simulink model "exo2_Part3_y"  (R2020b)
settings: Solver=VariableStepAuto  StartTime=0.0  StopTime=30.0  RelTol=1e-3
undefined symbols (not defined in the file or in its folder): fdesignblkfcn, gcbh
libraries: dspfdesign x4, vrlib x1
settings Model: Creator=elsibo  LastModifiedBy=YNS

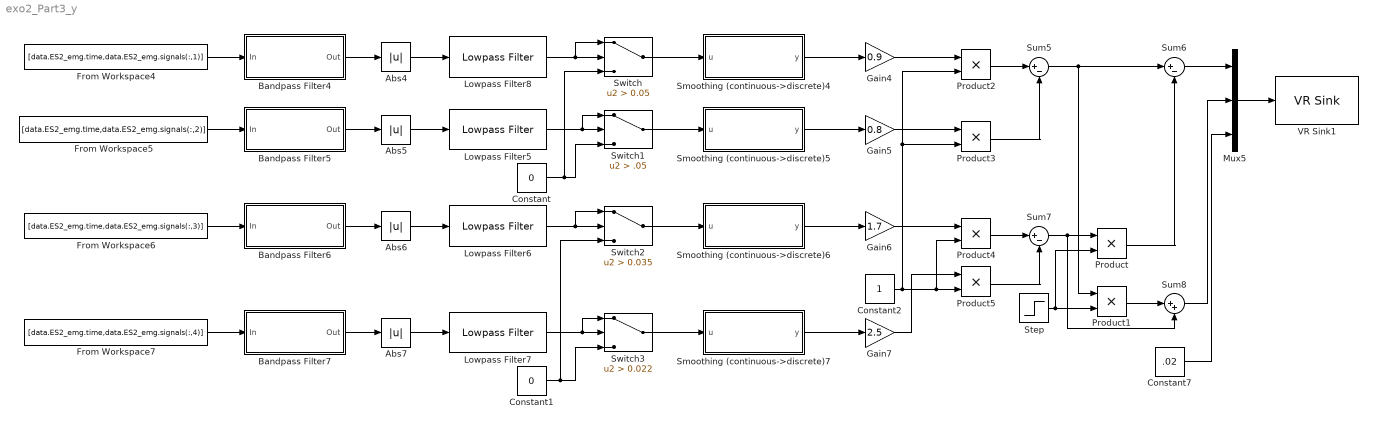
== system exo2_Part3_y ==
  Abs{4..7} (4 alike) : Abs
  Bandpass Filter4 : Subsystem  DialogController=fdesignblkfcn  InitFcn=fdesignblkfcn(gcbh, {'InitFcn'});  mask(Bandpass Filter){}
      mask help: Design a bandpass filter
      settings: CopyFcn=fdesignblkfcn(gcbh, {'CopyFcn'});
      mask Help: helpview(mapfilelocation('dsp'), 'dspbandpassfilter');
      mask Display: disp('Bandpass');
  Bandpass Filter5 : Subsystem  DialogController=fdesignblkfcn  InitFcn=fdesignblkfcn(gcbh, {'InitFcn'});  mask(Bandpass Filter){}
      mask help: Design a bandpass filter
      settings: CopyFcn=fdesignblkfcn(gcbh, {'CopyFcn'});
      mask Help: helpview(mapfilelocation('dsp'), 'dspbandpassfilter');
      mask Display: disp('Bandpass');
  Bandpass Filter6 : Subsystem  DialogController=fdesignblkfcn  InitFcn=fdesignblkfcn(gcbh, {'InitFcn'});  mask(Bandpass Filter){}
      mask help: Design a bandpass filter
      settings: CopyFcn=fdesignblkfcn(gcbh, {'CopyFcn'});
      mask Help: helpview(mapfilelocation('dsp'), 'dspbandpassfilter');
      mask Display: disp('Bandpass');
  Bandpass Filter7 : Subsystem  DialogController=fdesignblkfcn  InitFcn=fdesignblkfcn(gcbh, {'InitFcn'});  mask(Bandpass Filter){}
      mask help: Design a bandpass filter
      settings: CopyFcn=fdesignblkfcn(gcbh, {'CopyFcn'});
      mask Help: helpview(mapfilelocation('dsp'), 'dspbandpassfilter');
      mask Display: disp('Bandpass');
  Constant : Constant  Value=0
  Constant1 : Constant  Value=0
  Constant2 : Constant
  Constant7 : Constant  Value=.02
  From Workspace4 : FromWorkspace  VariableName=[data.ES2_emg.time,data.ES2_emg.signals(:,1)]  SampleTime=1/3000
  From Workspace5 : FromWorkspace  VariableName=[data.ES2_emg.time,data.ES2_emg.signals(:,2)]  SampleTime=1/3000
  From Workspace6 : FromWorkspace  VariableName=[data.ES2_emg.time,data.ES2_emg.signals(:,3)]  SampleTime=1/3000
  From Workspace7 : FromWorkspace  VariableName=[data.ES2_emg.time,data.ES2_emg.signals(:,4)]  SampleTime=1/3000
  Gain4 : Gain  Gain=0.9
  Gain5 : Gain  Gain=0.8
  Gain6 : Gain  Gain=1.7
  Gain7 : Gain  Gain=2.5
  Lowpass Filter5 : dspfdesign/Lowpass Filter  FilterType=FIR  DesignForMinimumOrder=on  FilterOrder=50  PassbandFrequency=3  StopbandFrequency=6  PassbandRipple=0.1  StopbandAttenuation=80  InheritSampleRate=off  SampleRate=1000  SimulateUsing=Interpreted execution  roundingMode=Floor  coeffsDataTypeStr=fixdt(1,16)
  Lowpass Filter6 : dspfdesign/Lowpass Filter  FilterType=FIR  DesignForMinimumOrder=on  FilterOrder=50  PassbandFrequency=3  StopbandFrequency=6  PassbandRipple=0.1  StopbandAttenuation=80  InheritSampleRate=off  SampleRate=1000  SimulateUsing=Interpreted execution  roundingMode=Floor  coeffsDataTypeStr=fixdt(1,16)
  Lowpass Filter7 : dspfdesign/Lowpass Filter  FilterType=FIR  DesignForMinimumOrder=on  FilterOrder=50  PassbandFrequency=3  StopbandFrequency=6  PassbandRipple=0.1  StopbandAttenuation=80  InheritSampleRate=off  SampleRate=1000  SimulateUsing=Interpreted execution  roundingMode=Floor  coeffsDataTypeStr=fixdt(1,16)
  Lowpass Filter8 : dspfdesign/Lowpass Filter  FilterType=FIR  DesignForMinimumOrder=on  FilterOrder=50  PassbandFrequency=3e3  StopbandFrequency=5e3  PassbandRipple=0.1  StopbandAttenuation=80  InheritSampleRate=off  SampleRate=44100  SimulateUsing=Interpreted execution  roundingMode=Floor  coeffsDataTypeStr=fixdt(1,16)
  Mux5 : Mux  Inputs=3
  Product{,1..5} (6 alike) : Product
  Smoothing (continuous->discrete)4 : Subsystem  mask(Smoothing (continuous->discrete)){tsSmoothing=0.35, smoothing0=0}
      mask prompts: tsSmoothing "physmod:simscape:couplers:SimscapeNetworkCouplersLib:SmoothingTimeConstants_MP"; smoothing0 "physmod:simscape:couplers:SimscapeNetworkCouplersLib:InitialOutput_MP"
      mask help: physmod:simscape:couplers:SimscapeNetworkCouplersLib:Smoothingcontinuousdiscrete_MD
      mask Help: web([docroot '/physmod/simscape/ref/networkcouplersmoothingcontinuousdiscrete.html'])
  Smoothing (continuous->discrete)5 : Subsystem  mask(Smoothing (continuous->discrete)){tsSmoothing=0.35, smoothing0=0}
      mask prompts: tsSmoothing "physmod:simscape:couplers:SimscapeNetworkCouplersLib:SmoothingTimeConstants_MP"; smoothing0 "physmod:simscape:couplers:SimscapeNetworkCouplersLib:InitialOutput_MP"
      mask help: physmod:simscape:couplers:SimscapeNetworkCouplersLib:Smoothingcontinuousdiscrete_MD
      mask Help: web([docroot '/physmod/simscape/ref/networkcouplersmoothingcontinuousdiscrete.html'])
  Smoothing (continuous->discrete)6 : Subsystem  mask(Smoothing (continuous->discrete)){tsSmoothing=0.35, smoothing0=0}
      mask prompts: tsSmoothing "physmod:simscape:couplers:SimscapeNetworkCouplersLib:SmoothingTimeConstants_MP"; smoothing0 "physmod:simscape:couplers:SimscapeNetworkCouplersLib:InitialOutput_MP"
      mask help: physmod:simscape:couplers:SimscapeNetworkCouplersLib:Smoothingcontinuousdiscrete_MD
      mask Help: web([docroot '/physmod/simscape/ref/networkcouplersmoothingcontinuousdiscrete.html'])
  Smoothing (continuous->discrete)7 : Subsystem  mask(Smoothing (continuous->discrete)){tsSmoothing=0.35, smoothing0=0}
      mask prompts: tsSmoothing "physmod:simscape:couplers:SimscapeNetworkCouplersLib:SmoothingTimeConstants_MP"; smoothing0 "physmod:simscape:couplers:SimscapeNetworkCouplersLib:InitialOutput_MP"
      mask help: physmod:simscape:couplers:SimscapeNetworkCouplersLib:Smoothingcontinuousdiscrete_MD
      mask Help: web([docroot '/physmod/simscape/ref/networkcouplersmoothingcontinuousdiscrete.html'])
  Step : Step  Time=15  SampleTime=0
  Sum5 : Sum  Inputs=|+-
  Sum6 : Sum  Inputs=|+-
  Sum7 : Sum  Inputs=|+-
  Sum8 : Sum  Inputs=|++
  Switch : Switch  Criteria=u2 > Threshold  Threshold=0.05
  Switch1 : Switch  Criteria=u2 > Threshold  Threshold=.05
  Switch2 : Switch  Criteria=u2 > Threshold  Threshold=0.035
  Switch3 : Switch  Criteria=u2 > Threshold  Threshold=0.022
  VR Sink1 : vrlib/VR Sink  InstantiateOnLoad=on  SampleTime=0.1  ViewEnable=on  RemoteChange=off  RemoteView=off  FieldsWritten=cursor.translation.3.1.1.double  WorldFileName=8_palline_color.wrl  AutoView=off  VideoDimensions=[]  AllowVariableSize=off
  wires:
  Constant2/1 -> Product4/2, Product5/2, Product2/2, Product3/2
  Bandpass Filter6/1(Out) -> Abs6/1
  Bandpass Filter5/1(Out) -> Abs5/1
  Product2/1 -> Sum5/1
  From Workspace4/1 -> Bandpass Filter4/1(In)
  Bandpass Filter4/1(Out) -> Abs4/1
  Sum7/1 -> Sum8/2, Product/1
  Product4/1 -> Sum7/1
  From Workspace5/1 -> Bandpass Filter5/1(In)
  From Workspace7/1 -> Bandpass Filter7/1(In)
  Gain7/1 -> Product5/1
  Abs4/1 -> Lowpass Filter8/1
  Bandpass Filter7/1(Out) -> Abs7/1
  Sum6/1 -> Mux5/1
  From Workspace6/1 -> Bandpass Filter6/1(In)
  Abs5/1 -> Lowpass Filter5/1
  Abs6/1 -> Lowpass Filter6/1
  Gain6/1 -> Product4/1
  Constant/1 -> Switch/3, Switch1/3
  Abs7/1 -> Lowpass Filter7/1
  Smoothing (continuous->discrete)6/1(y) -> Gain6/1
  Lowpass Filter8/1 -> Switch/1, Switch/2
  Lowpass Filter5/1 -> Switch1/1, Switch1/2
  Lowpass Filter6/1 -> Switch2/2, Switch2/1
  Lowpass Filter7/1 -> Switch3/1, Switch3/2
  Gain5/1 -> Product3/1
  Switch2/1 -> Smoothing (continuous->discrete)6/1(u)
  Constant1/1 -> Switch2/3, Switch3/3
  Switch/1 -> Smoothing (continuous->discrete)4/1(u)
  Product5/1 -> Sum7/2
  Switch1/1 -> Smoothing (continuous->discrete)5/1(u)
  Switch3/1 -> Smoothing (continuous->discrete)7/1(u)
  Smoothing (continuous->discrete)4/1(y) -> Gain4/1
  Smoothing (continuous->discrete)5/1(y) -> Gain5/1
  Smoothing (continuous->discrete)7/1(y) -> Gain7/1
  Mux5/1 -> VR Sink1/1
  Constant7/1 -> Mux5/3
  Gain4/1 -> Product2/1
  Product3/1 -> Sum5/2
  Step/1 -> Product1/2, Product/2
  Sum5/1 -> Sum6/1, Product1/1
  Sum8/1 -> Mux5/2
  Product1/1 -> Sum8/1
  Product/1 -> Sum6/2

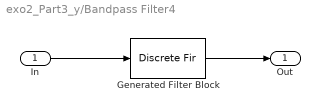
== system exo2_Part3_y/Bandpass Filter4 ==
  In : Inport
  Generated Filter Block : DiscreteFir  Tag=BlockMethodSubSystem  Coefficients=[0.0247784165301608433 0.00982645761123041028 -0.076956364309928485 -0.00574234407939242311 -0.0280411528162793217 -0.00804608705322140162 -0.0118695570715928369 -0.00997698951682126148 -0.0032900682882155835 -0.0123964456094048502 0.00352600878115876329 -0.0139189700142880405 0.00905023941727317073 -0.0130997642055635105 0.0124656128815527987 -0.00909287544946293935 0.0131317697099942975 -0.00207947540041804888 0.0111769210630364487 0.00659009778413368903 0.00765273613394504455 0.0147232835745342554 0.00427867752512019368 0.0199633122366019398 0.00267711132018813233 0.0203811397583988814 0.0037418940950067715 0.0149169811807585064 0.00742876303379174253 0.00413015922899517742 0.0123258049521986213 -0.00967745920215465696 0.015760250203825283 -0.0236422789640416652 0.0148621759121691233 -0.0338874815186639144 0.00685197471547598861 -0.0377812878977663025 -0.00958300552505572667 -0.0336540649346103726 -0.0340410723239205834 -0.0220502805385552648 -0.063942206809497748 -0.00527010472050306374 -0.0951066582635559377 0.0128546225834283885 -0.12245473858081414 0.0280548282114237782 -0.141172435722598355 0.0367254315914400456 0.852170468203800047 0.0367254315914400456 -0.141172435722598355 0.0280548282114237782 -0.12245473858081414 0.0128546225834283885 -0.0951066582635559377 -0.00527010472050306374 -0.063942206809497748 -0.0220502805385552648 -0.0340410723239205834 -0.0336540649346103726 -0.00958300552505572667 -0.0377812878977663025 0.00685197471547598861 -0.0338874815186639144 0.0148621759121691233 -0.0236422789640416652 0.015760250203825283 -0.00967745920215465696 0.0123258049521986213 0.00413015922899517742 0.00742876303379174253 0.0149169811807585064 0.0037418940950067715 0.0203811397583988814 0.00267711132018813233 0.0199633122366019398 0.00427867752512019368 0.0147232835745342554 0.00765273613394504455 0.00659009778413368903 0.0111769210630364487 -0.00207947540041804888 0.0131317697099942975 -0.00909287544946293935 0.0124656128815527987 -0.0130997642055635105 0.00905023941727317073 -0.0139189700142880405 0.00352600878115876329 -0.0123964456094048502 -0.0032900682882155835 -0.00997698951682126148 -0.0118695570715928369 -0.00804608705322140162 -0.0280411528162793217 -0.00574234407939242311 -0.076956364309928485 0.00982645761123041028 0.0247784165301608433]  InputProcessing=Columns as channels (frame based)
  Out : Outport  VectorParamsAs1DForOutWhenUnconnected=off
  wires:
  In/1 -> Generated Filter Block/1
  Generated Filter Block/1 -> Out/1

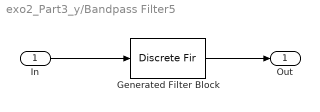
== system exo2_Part3_y/Bandpass Filter5 ==
  In : Inport
  Generated Filter Block : DiscreteFir  Tag=BlockMethodSubSystem  Coefficients=[0.0247784165301608433 0.00982645761123041028 -0.076956364309928485 -0.00574234407939242311 -0.0280411528162793217 -0.00804608705322140162 -0.0118695570715928369 -0.00997698951682126148 -0.0032900682882155835 -0.0123964456094048502 0.00352600878115876329 -0.0139189700142880405 0.00905023941727317073 -0.0130997642055635105 0.0124656128815527987 -0.00909287544946293935 0.0131317697099942975 -0.00207947540041804888 0.0111769210630364487 0.00659009778413368903 0.00765273613394504455 0.0147232835745342554 0.00427867752512019368 0.0199633122366019398 0.00267711132018813233 0.0203811397583988814 0.0037418940950067715 0.0149169811807585064 0.00742876303379174253 0.00413015922899517742 0.0123258049521986213 -0.00967745920215465696 0.015760250203825283 -0.0236422789640416652 0.0148621759121691233 -0.0338874815186639144 0.00685197471547598861 -0.0377812878977663025 -0.00958300552505572667 -0.0336540649346103726 -0.0340410723239205834 -0.0220502805385552648 -0.063942206809497748 -0.00527010472050306374 -0.0951066582635559377 0.0128546225834283885 -0.12245473858081414 0.0280548282114237782 -0.141172435722598355 0.0367254315914400456 0.852170468203800047 0.0367254315914400456 -0.141172435722598355 0.0280548282114237782 -0.12245473858081414 0.0128546225834283885 -0.0951066582635559377 -0.00527010472050306374 -0.063942206809497748 -0.0220502805385552648 -0.0340410723239205834 -0.0336540649346103726 -0.00958300552505572667 -0.0377812878977663025 0.00685197471547598861 -0.0338874815186639144 0.0148621759121691233 -0.0236422789640416652 0.015760250203825283 -0.00967745920215465696 0.0123258049521986213 0.00413015922899517742 0.00742876303379174253 0.0149169811807585064 0.0037418940950067715 0.0203811397583988814 0.00267711132018813233 0.0199633122366019398 0.00427867752512019368 0.0147232835745342554 0.00765273613394504455 0.00659009778413368903 0.0111769210630364487 -0.00207947540041804888 0.0131317697099942975 -0.00909287544946293935 0.0124656128815527987 -0.0130997642055635105 0.00905023941727317073 -0.0139189700142880405 0.00352600878115876329 -0.0123964456094048502 -0.0032900682882155835 -0.00997698951682126148 -0.0118695570715928369 -0.00804608705322140162 -0.0280411528162793217 -0.00574234407939242311 -0.076956364309928485 0.00982645761123041028 0.0247784165301608433]  InputProcessing=Columns as channels (frame based)
  Out : Outport  VectorParamsAs1DForOutWhenUnconnected=off
  wires:
  In/1 -> Generated Filter Block/1
  Generated Filter Block/1 -> Out/1

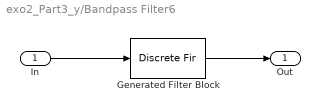
== system exo2_Part3_y/Bandpass Filter6 ==
  In : Inport
  Generated Filter Block : DiscreteFir  Tag=BlockMethodSubSystem  Coefficients=[0.0247784165301608433 0.00982645761123041028 -0.076956364309928485 -0.00574234407939242311 -0.0280411528162793217 -0.00804608705322140162 -0.0118695570715928369 -0.00997698951682126148 -0.0032900682882155835 -0.0123964456094048502 0.00352600878115876329 -0.0139189700142880405 0.00905023941727317073 -0.0130997642055635105 0.0124656128815527987 -0.00909287544946293935 0.0131317697099942975 -0.00207947540041804888 0.0111769210630364487 0.00659009778413368903 0.00765273613394504455 0.0147232835745342554 0.00427867752512019368 0.0199633122366019398 0.00267711132018813233 0.0203811397583988814 0.0037418940950067715 0.0149169811807585064 0.00742876303379174253 0.00413015922899517742 0.0123258049521986213 -0.00967745920215465696 0.015760250203825283 -0.0236422789640416652 0.0148621759121691233 -0.0338874815186639144 0.00685197471547598861 -0.0377812878977663025 -0.00958300552505572667 -0.0336540649346103726 -0.0340410723239205834 -0.0220502805385552648 -0.063942206809497748 -0.00527010472050306374 -0.0951066582635559377 0.0128546225834283885 -0.12245473858081414 0.0280548282114237782 -0.141172435722598355 0.0367254315914400456 0.852170468203800047 0.0367254315914400456 -0.141172435722598355 0.0280548282114237782 -0.12245473858081414 0.0128546225834283885 -0.0951066582635559377 -0.00527010472050306374 -0.063942206809497748 -0.0220502805385552648 -0.0340410723239205834 -0.0336540649346103726 -0.00958300552505572667 -0.0377812878977663025 0.00685197471547598861 -0.0338874815186639144 0.0148621759121691233 -0.0236422789640416652 0.015760250203825283 -0.00967745920215465696 0.0123258049521986213 0.00413015922899517742 0.00742876303379174253 0.0149169811807585064 0.0037418940950067715 0.0203811397583988814 0.00267711132018813233 0.0199633122366019398 0.00427867752512019368 0.0147232835745342554 0.00765273613394504455 0.00659009778413368903 0.0111769210630364487 -0.00207947540041804888 0.0131317697099942975 -0.00909287544946293935 0.0124656128815527987 -0.0130997642055635105 0.00905023941727317073 -0.0139189700142880405 0.00352600878115876329 -0.0123964456094048502 -0.0032900682882155835 -0.00997698951682126148 -0.0118695570715928369 -0.00804608705322140162 -0.0280411528162793217 -0.00574234407939242311 -0.076956364309928485 0.00982645761123041028 0.0247784165301608433]  InputProcessing=Columns as channels (frame based)
  Out : Outport  VectorParamsAs1DForOutWhenUnconnected=off
  wires:
  In/1 -> Generated Filter Block/1
  Generated Filter Block/1 -> Out/1

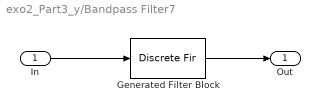
== system exo2_Part3_y/Bandpass Filter7 ==
  In : Inport
  Generated Filter Block : DiscreteFir  Tag=BlockMethodSubSystem  Coefficients=[0.0247784165301608433 0.00982645761123041028 -0.076956364309928485 -0.00574234407939242311 -0.0280411528162793217 -0.00804608705322140162 -0.0118695570715928369 -0.00997698951682126148 -0.0032900682882155835 -0.0123964456094048502 0.00352600878115876329 -0.0139189700142880405 0.00905023941727317073 -0.0130997642055635105 0.0124656128815527987 -0.00909287544946293935 0.0131317697099942975 -0.00207947540041804888 0.0111769210630364487 0.00659009778413368903 0.00765273613394504455 0.0147232835745342554 0.00427867752512019368 0.0199633122366019398 0.00267711132018813233 0.0203811397583988814 0.0037418940950067715 0.0149169811807585064 0.00742876303379174253 0.00413015922899517742 0.0123258049521986213 -0.00967745920215465696 0.015760250203825283 -0.0236422789640416652 0.0148621759121691233 -0.0338874815186639144 0.00685197471547598861 -0.0377812878977663025 -0.00958300552505572667 -0.0336540649346103726 -0.0340410723239205834 -0.0220502805385552648 -0.063942206809497748 -0.00527010472050306374 -0.0951066582635559377 0.0128546225834283885 -0.12245473858081414 0.0280548282114237782 -0.141172435722598355 0.0367254315914400456 0.852170468203800047 0.0367254315914400456 -0.141172435722598355 0.0280548282114237782 -0.12245473858081414 0.0128546225834283885 -0.0951066582635559377 -0.00527010472050306374 -0.063942206809497748 -0.0220502805385552648 -0.0340410723239205834 -0.0336540649346103726 -0.00958300552505572667 -0.0377812878977663025 0.00685197471547598861 -0.0338874815186639144 0.0148621759121691233 -0.0236422789640416652 0.015760250203825283 -0.00967745920215465696 0.0123258049521986213 0.00413015922899517742 0.00742876303379174253 0.0149169811807585064 0.0037418940950067715 0.0203811397583988814 0.00267711132018813233 0.0199633122366019398 0.00427867752512019368 0.0147232835745342554 0.00765273613394504455 0.00659009778413368903 0.0111769210630364487 -0.00207947540041804888 0.0131317697099942975 -0.00909287544946293935 0.0124656128815527987 -0.0130997642055635105 0.00905023941727317073 -0.0139189700142880405 0.00352600878115876329 -0.0123964456094048502 -0.0032900682882155835 -0.00997698951682126148 -0.0118695570715928369 -0.00804608705322140162 -0.0280411528162793217 -0.00574234407939242311 -0.076956364309928485 0.00982645761123041028 0.0247784165301608433]  InputProcessing=Columns as channels (frame based)
  Out : Outport  VectorParamsAs1DForOutWhenUnconnected=off
  wires:
  In/1 -> Generated Filter Block/1
  Generated Filter Block/1 -> Out/1

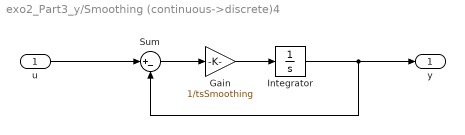
== system exo2_Part3_y/Smoothing (continuous->discrete)4 ==
  u : Inport
  Gain : Gain  Gain=1/tsSmoothing
  Integrator : Integrator  InitialCondition=smoothing0
  Sum : Sum  Inputs=|+-
  y : Outport
  wires:
  u/1 -> Sum/1
  Integrator/1 -> Sum/2, y/1
  Gain/1 -> Integrator/1
  Sum/1 -> Gain/1

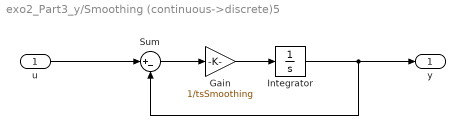
== system exo2_Part3_y/Smoothing (continuous->discrete)5 ==
  u : Inport
  Gain : Gain  Gain=1/tsSmoothing
  Integrator : Integrator  InitialCondition=smoothing0
  Sum : Sum  Inputs=|+-
  y : Outport
  wires:
  u/1 -> Sum/1
  Integrator/1 -> Sum/2, y/1
  Gain/1 -> Integrator/1
  Sum/1 -> Gain/1

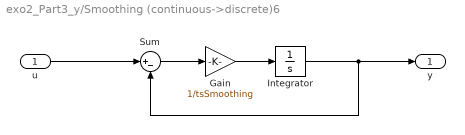
== system exo2_Part3_y/Smoothing (continuous->discrete)6 ==
  u : Inport
  Gain : Gain  Gain=1/tsSmoothing
  Integrator : Integrator  InitialCondition=smoothing0
  Sum : Sum  Inputs=|+-
  y : Outport
  wires:
  u/1 -> Sum/1
  Integrator/1 -> Sum/2, y/1
  Gain/1 -> Integrator/1
  Sum/1 -> Gain/1

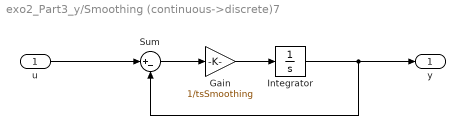
== system exo2_Part3_y/Smoothing (continuous->discrete)7 ==
  u : Inport
  Gain : Gain  Gain=1/tsSmoothing
  Integrator : Integrator  InitialCondition=smoothing0
  Sum : Sum  Inputs=|+-
  y : Outport
  wires:
  u/1 -> Sum/1
  Integrator/1 -> Sum/2, y/1
  Gain/1 -> Integrator/1
  Sum/1 -> Gain/1
